simulink model "uz_ParameterID6ph"  (R2021b)
settings: Solver=FixedStepDiscrete  StartTime=0.0  StopTime=160  FixedStep=0.000005  RelTol=1e-3  EnableMultiTasking=on
model workspace (MATLAB code in the model file):
  | cmdLim = Simulink.Parameter;
  | cmdLim.Value = 15;
  | cmdLim.Description = 'Limit for controlling the maximum surface command angle.';
  | cmdLim.Min = 0;
  | cmdLim.Max = 90;
  | cmdLim.DocUnits = 'deg';
  | 
  | dispGain = Simulink.Parameter;
  | dispGain.Value = 0.75;
  | dispGain.Description = 'Gain applied to the displacement error.';
  | dispGain.Min = 0;
  | dispGain.Max = [];
  | dispGain.DocUnits = 'deg/sec/deg';
  | 
  | dispLim = Simulink.Parameter;
  | dispLim.Value = 30;
  | dispLim.Description = 'Limit for controlling the maximum commanded angle.';
  | dispLim.Min = 0;
  | dispLim.Max = 180;
  | dispLim.DocUnits = 'deg';
  | 
  | intGain = Simulink.Parameter;
  | intGain.Value = 0.5;
  | intGain.Description = 'Gain applied to the integral error.';
  | intGain.Min = 0;
  | intGain.Max = [];
  | intGain.DocUnits = 'deg/sec/deg/sec';
  | 
  | intLim = Simulink.Parameter;
  | intLim.Value = 5;
  | intLim.Description = 'Limit for controlling the maximum commanded angle.';
  | intLim.Min = 0;
  | intLim.Max = 90;
  | intLim.DocUnits = 'deg';
  | 
  | rateGain = Simulink.Parameter;
  | rateGain.Value = 2;
  | rateGain.Description = 'Gain applied to the rate error.';
  | rateGain.Min = 0;
  | rateGain.Max = [];
  | rateGain.DocUnits = 'deg/deg/sec';
  | 
  | rateLim = Simulink.Parameter;
  | rateLim.Value = 6;
  | rateLim.Description = 'Limit for controlling the maximum commanded angle.';
  | rateLim.Min = 0;
  | rateLim.Max = 180;
  | rateLim.DocUnits = 'deg/sec';
  | 
  | hdgGain = Simulink.Parameter;
  | hdgGain.Value = 0.015;
values from neighbouring files (symbols this model uses):
  c = 2/6*cat(1,tl1,tl2,tl3,tl4,tl5,tl6)    [Parameter_Init_Buehler_201_6ph.m]
  d_d_TMS = 0.005    [Parameter_Init_Buehler_201.m]
  d_f_hardware = 200000    [Parameter_Init_Buehler_201.m]
  d_f_states = 20000    [Parameter_Init_Buehler_201.m]
  d_i_max = 15    [Parameter_Init_Buehler_201.m]
  d_i_min = -d_i_max    (= -15)    [Parameter_Init_Buehler_201.m]
  d_I_n = 8    [Parameter_Init_Buehler_201.m]
  d_J_Coupling_M_E = 2e-6    (= 2e-06)    [Parameter_Init_Buehler_201.m]
  d_J_Coupling_M_Ms = 2e-20    [Parameter_Init_Buehler_201.m]
  d_J_Ms_L = d_J_Ms_M    (= 1.26363648e-05)    [Parameter_Init_Buehler_201.m]
  d_J_Ms_M = 0.5*0.5*((0.5*d_d_Ms)^4)*3.14*d_l_Ms*d_rho_Ms    (= 1.26363648e-05)    [Parameter_Init_Buehler_201.m]
  d_Ki_id = 162.47    [Parameter_Init_Buehler_201.m]
  d_Ki_iq = 162.47    [Parameter_Init_Buehler_201.m]
  d_Ki_n = 1.982    [Parameter_Init_Buehler_201.m]
  d_Kp_id = 0.369    [Parameter_Init_Buehler_201.m]
  d_Kp_iq = 0.369    [Parameter_Init_Buehler_201.m]
  d_Kp_n = 0.198    [Parameter_Init_Buehler_201.m]
  d_L_d = 0.00031    [Parameter_Init_Buehler_201.m]
  d_L_q = 0.00033    [Parameter_Init_Buehler_201.m]
  d_n_n = 3200    [Parameter_Init_Buehler_201.m]
  d_p = 4    [Parameter_Init_Buehler_201.m]
  d_psi_pm = 0.0075    [Parameter_Init_Buehler_201.m]
  d_R_ph = d_R_ph_ph/2    (= 0.089)    [Parameter_Init_Buehler_201.m]
  d_y_max = 10    [Parameter_Init_Buehler_201.m]
  d_y_min = -d_y_max    (= -10)    [Parameter_Init_Buehler_201.m]
  V_DC = 24    [Parameter_Init_Buehler_201.m]
undefined symbols (not defined in the file or in its folder): i_dq, i_dq_ref, n_ref, ts_ps, V_abc, v_dq
libraries: fl_lib x66, nesl_utility x51, ee_lib x38, simulink x14, spsTriangleGeneratorLib x3, spsabctodq0Lib x2, spsAlphaBetaZerotodq0Lib x2, spsdq0toabcLib x1
(part 6 of 6)

== matlab function uz_ParameterID6ph/CleanPsiArray ==
  data: OnlineID_output input; psi_array_out output; eta_c input; array_cleaned_flag output boolean; n_flux_points output
function [psi_array_out,array_cleaned_flag,n_flux_points]=clean_psi_array(OnlineID_output,eta_c)
% Author Philipp Gebhardt
% Oktober 2019

%This function is cleaning the array storing the measurement values, which always consits of a d-q-current combination a winding temperature and a speed value such as a d-q-flux combination
%The function is searching for measuring pairs which are closer than eta_c to their neighbours. In this case it is averaging these similar pairs to avoid measuring values storing the same information. 
%This is essential for calculating a wide ranging flux maps out of this array.
%Furthermore there is an output n_flux_points giving back the amount of independent measuring pairs


%Initialising Outputs
n_flux_points=single(1);
psi_array_out=single(zeros(6,100));
clean_curr_count=single(0);
array_cleaned_flag=boolean(0);

if(OnlineID_output.clean_array == 1)
% Searching for similar Datapairs
for(k=single(1):single(length(OnlineID_output.psi_array(1,:))))
    eta_count=0;
   
    if (OnlineID_output.psi_array(3,k)~=0)
        for(t=single(1):single(length(OnlineID_output.psi_array(1,:))))
            if (OnlineID_output.psi_array(3,t)~=0)
                if(k<t)    
                    if( (    (OnlineID_output.psi_array(1,k)-OnlineID_output.psi_array(1,t))^2  +...
                        (OnlineID_output.psi_array(2,k)-OnlineID_output.psi_array(2,t))^2     )^0.5 < eta_c )       
        %Averaging Datapairs if they are to close to each other
        
                        OnlineID_output.psi_array(1,t)=(OnlineID_output.psi_array(1,k)+OnlineID_output.psi_array(1,t))*0.5;
                        OnlineID_output.psi_array(2,t)=(OnlineID_output.psi_array(2,k)+OnlineID_output.psi_array(2,t))*0.5;
                        OnlineID_output.psi_array(3,t)=(OnlineID_output.psi_array(3,k)+OnlineID_output.psi_array(3,t))*0.5;
                        OnlineID_output.psi_array(4,t)=(OnlineID_output.psi_array(4,k)+OnlineID_output.psi_array(4,t))*0.5;                    
                        OnlineID_output.psi_array(5,t)=(OnlineID_output.psi_array(5,k)+OnlineID_output.psi_array(5,t))*0.5;
                        OnlineID_output.psi_array(6,t)=(OnlineID_output.psi_array(6,k)+OnlineID_output.psi_array(6,t))*0.5;     
                        OnlineID_output.psi_array(1:6,k)=0;
                        eta_count=1;  
                    end    
                end
            end
     
            if eta_count==1
                break
            end     
        end 
            if(eta_count==0)       
                %Accept values if there is enough distance between them
                clean_curr_count=clean_curr_count+1;
                psi_array_out(1,clean_curr_count)=OnlineID_output.psi_array(1,k);
                psi_array_out(2,clean_curr_count)=OnlineID_output.psi_array(2,k);
                psi_array_out(3,clean_curr_count)=OnlineID_output.psi_array(3,k);
                psi_array_out(4,clean_curr_count)=OnlineID_output.psi_array(4,k);
                psi_array_out(5,clean_curr_count)=OnlineID_output.psi_array(5,k);
                psi_array_out(6,clean_curr_count)=OnlineID_output.psi_array(6,k);
            end
    end
end

% Count flux points
for(k=single(1):single(length(psi_array_out(1,:))))  
    if(psi_array_out(1,k)~=0||psi_array_out(2,k)~=0||psi_array_out(3,k)~=0)       
           n_flux_points=k;
    end    
end

array_cleaned_flag=boolean(1);
end
return;

== matlab function uz_ParameterID6ph/dqTrans/VoltageTransformation/Filterkorrektur_Hardware ==
  data: phi output; u input; y output; omega input; phi input

function [phi,y]= fcn(u,omega, phi)

R=95300;%ohm
RL=8200;%ohm
C=0.000000047;%Farrad
T=(RL*R*C)/(R+RL);

 w=omega;
%Filter zur Kompensation des Phasenversatz der Spannungen
 for i=single(1):single(3)
     %Rückgängigkmachen der ADC Umrechung und umkehren der Filterfunktion
u(i)=u(i)*(1+( w*T)^2)^0.5;
 end
 

phi=(phi)- atan(  w*T   );%atan(  w*T   );%*(1.08);


y = u;

== matlab function uz_ParameterID6ph/FOC/Space vector limitation ==
  data: v_d_limit output; v_q_limit output; ActualValues input; v_d_in input single; v_q_in input; limit_on output boolean
% Algorithm for voltage space vector limitation
% 
% Quelle:    Vector Control of Three-Phase AC Machines, S. 183
% Autoren:   Nguyen Phung Quang, Jörg-Andreas Dittrich
%            Springer, 2015,Second Edition


function [v_d_limit, v_q_limit,limit_on] = fcn(ActualValues,v_d_in, v_q_in)
% max amplitude of the space vectors
   % with addition of 3rd harmonics   U^_LN = V_DC/2;
   %V_DC_max = V_DC*0.5;
   %with offset addition of 3rd harmonics  V^_LN = V_DC/sqrt(3);
   V_SV_max =ActualValues.V_DC/sqrt(3);

% absolue value of the space vector from vd and vq
V_SV_abs = sqrt(v_d_in^2 + v_q_in^2);

% limitation necessary?
if ( V_SV_abs > V_SV_max )   
    limit_on = boolean(1);   % limitation is necessary -> generator or drive operation?
   
    if ((sign(ActualValues.omega_el)==sign(ActualValues.i_dq.q)) ) % drive operation      
        Error = 0;
        if ( (abs(v_d_in) > 0.95*V_SV_max) )
        %true
        v_d_limit = sign(v_d_in)*0.95*V_SV_max;
        v_q_limit = sign(v_q_in)*sqrt(V_SV_max^2-v_d_limit^2);
        Fall = 2;
        else
        %false
        v_d_limit = v_d_in;
        v_q_limit = sign(v_q_in)*sqrt(V_SV_max^2-v_d_limit^2);
        Fall = 1;
        end    
    
    
    elseif ((sign(ActualValues.omega_el)~=sign(ActualValues.i_dq.q)) ) % generator operation   
        Error = 0;
        if ( abs(v_q_in) > 0.95*V_SV_max )
        %true
        v_q_limit = sign(v_q_in)*0.95*V_SV_max;
        v_d_limit = sign(v_d_in)*sqrt(V_SV_max^2-v_q_limit^2);
        %v_d_limit = U_d;        Fall = 4;       
        else 
        % false
        v_q_limit = v_q_in;
        v_d_limit = sign(v_d_in)*sqrt(V_SV_max^2-v_q_limit^2);
        Fall = 3;
        end
        
    else % Error
    v_d_limit = v_d_in;
    v_q_limit = v_q_in;
    Error = 1;
    Fall = 5;
    end
    
else
% no limitation necessary
    v_d_limit = v_d_in;
    v_q_limit = v_q_in;
    limit_on = boolean(0);
    Error = 0;
    Fall = 0;
end

v_d_in = v_d_limit;
v_q_in = v_q_limit;
end

== matlab function uz_ParameterID6ph/FOC/uz_FOC_Speed/Field Weakening/MATLAB Function ==
  data: I_max input single; id_soll output single; V_DC input single; R input single; Lq input single; Ld input single; psi_pm input single; omega_el input single; iq_max output; id_ref_input input
function [id_soll, iq_max]= field_weakening(I_max, V_DC, R, Lq, Ld, psi_pm, omega_el,id_ref_input)

%Maximum voltage vector
v_max_dq = single(0.95* V_DC/sqrt(single(3)));
fw_flag = boolean(0);
%Calculation of n_cut
a = single(I_max^2 * Lq^2 + psi_pm^2);
b = single(2*R*psi_pm*I_max);
c = single((I_max^2 * R^2)-v_max_dq^2);

omega_cut = single((-b + sqrt(b^2 - 4*a*c))/(2*a));


%Check if w_cut is valid
if omega_cut > 0 && isreal(single(omega_cut))  
    %Calcultation of Id_ref
    if omega_el > omega_cut
        fw_flag = boolean(1);
        id_ref_fw = single(psi_pm/Ld * (omega_cut/omega_el -1));
        if id_ref_fw < -I_max
            id_ref_fw = -I_max;
        end
    else
        id_ref_fw = single(0.0);
    end
else
    id_ref_fw = single(0.0);
end

if fw_flag == boolean(0)
    id_soll = single(id_ref_input);
elseif (fw_flag == boolean(1)) && (id_ref_input <= id_ref_fw)
    id_soll = single(id_ref_input);
else
    id_soll = single(id_ref_fw);
end

if id_soll < single(0.0)
   a_fw = single(R^2 + omega_el^2 * Lq^2);
   b_fw = single(2*R*omega_el*psi_pm);
   c_fw = single(id_soll^2 * R^2 -v_max_dq^2 + omega_el^2 * (psi_pm^2 + Ld^2 * id_soll^2 + 2*psi_pm*Ld*id_soll));
   
   iq_max = single((-b_fw + sqrt(b_fw^2 - 4*a_fw*c_fw))/(2*a_fw));
   if iq_max > single(sqrt(I_max^2 - id_soll^2))
      iq_max =  single(sqrt(I_max^2 - id_soll^2));
   end
else
    iq_max = single(sqrt(I_max^2 - id_soll^2));
end
